simulink model "xmc_fir_import"  (R2023a)
settings: Solver=VariableStepAuto  StartTime=0.0  StopTime=inf  RelTol=1e-3
PostLoadFcn:
  | xmcHubUpdateInstalledDevice(gcs);
undefined symbols (not defined in the file): xc7vx485tffg1157
libraries: vmcUtilities x2, hlsBasic x2, dspsrcs4 x1, fir_c_import x1
settings Model: Creator=abehbood  LastModifiedBy=robg
settings SolverCC: AlgebraicLoopSolver=TrustRegion
settings DataIOCC: ReturnWorkspaceOutputs=off
settings OptimizationCC: LifeSpan=inf
settings DebuggingCC: UnconnectedInputMsg=warning  UnconnectedOutputMsg=warning  UnconnectedLineMsg=warning  ArithmeticOperatorsInVariantConditions=warning
settings ModelReferenceCC: EnableRefExpFcnMdlSchedulingChecks=on
settings SFSimCC: SimUseLocalCustomCode=off  CustomCodeUndefinedFunction=UseInterfaceOnly
settings RTWCC: RTWUseLocalCustomCode=off  DLArmComputeVersion=19.05
settings CodeAppCC: StateflowObjectComments=on

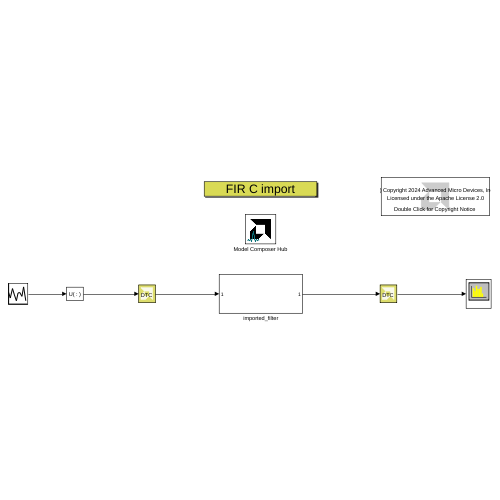
[thumbnail: Simulink's stored preview of the top-level diagram]
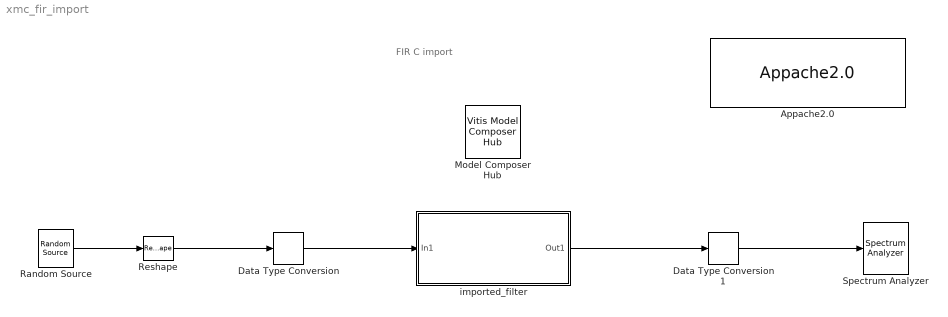
== system xmc_fir_import ==
  note: FIR C import
  Appache2.0 : vmcUtilities/Appache2.0
  Data Type Conversion : hlsBasic/Data Type Conversion  OutDataType=fixed  TypeExp=''  Signedness=Signed  WordLength=17  FractionalLength=14  RoundingMode=Truncation to minus infinity  OverflowMode=Wrap around
  Data Type Conversion1 : hlsBasic/Data Type Conversion  OutDataType=double  TypeExp=''  Signedness=Signed  WordLength=16  FractionalLength=0  RoundingMode=Truncation to minus infinity  OverflowMode=Wrap around
  Model Composer Hub : vmcUtilities/Vitis Model Composer Hub  Tag=genX  CodeGeneration=off  SubsystemName=imported_filter  StartColumn=1  NumberOfColumns=1  TargetDirectory=./code  exportDesign=off  analyzeDesign=off  validateDesignOnHw=off  ExportType=HLS C++ code  IpVendor=xilinx.com  IpLibrary=hls  IpVersion=1.0  IpHWLanguage=Verilog  AieCompilerOptions={}  AieSimulatorOptions={}  CreateTestbench=off  TestbenchStackSize=10  RunRtlSim=off  RunCSim=off  RunAieSim=off  AieSimTimeout=50000  RunAieSimProfiling=off  LaunchVitisAnalyzer=off  PlotOutput=off  RunX86Sim=on  X86SimTimeout=10  GenHwImage=off  GenLibadfXo=off  GenHwValidationCode=off  PlatformType=Not Specified  HwSystemType=Baremetal  HwValidationTarget=hw  ProjDevice=xc7vx485tffg1157-1  ProjDevicePart=xc7vx485tffg1157-1  SamplePeriod=-1  ClockFrequency=200  DataPathParallelism=1  xilinxfamily=Kintex7  part=xc7k325t  speed=-3  package=fbg676  directory=./netlist  testbench=off  incr_netlist=off  synthesis_tool=Vivado  clock_wrapper=Clock Enables  dbl_ovrd=According to Block Masks  dcm_input_clock_period=10  sysclk_period=10  simulink_period=1  eval_field=0  LogFileName=''  NThreads=4
  Random Source : dspsrcs4/Random Source  SrcType=Gaussian  NormMethod=Ziggurat  CltLength=12  MinVal=0  MaxVal=1  MeanVal=0  VarVal=1  RepMode=Not repeatable  rawSeed=1  IsInherit=off  SampMode=Discrete  SampTime=1  SampFrame=100  DataType=Double  OutComplex=Real  OutputFrames=off
  Reshape : Reshape
  Spectrum Analyzer : SpectrumAnalyzer  WindowPosition=[506 197 832 446]  Method=Welch  SampleRate=1  Span=1  StartFrequency=-0.5  StopFrequency=0.5  AveragingMethod=Exponential  YLimits=[-112.1969,21.3448]  ChannelNames="[\"\"]"  DefaultConfigurationName=spbscopes.SpectrumAnalyzerBlockCfg
  imported_filter : Subsystem
  wires:
  Data Type Conversion1/1 -> Spectrum Analyzer/1
  Random Source/1 -> Reshape/1
  Data Type Conversion/1 -> imported_filter/1(In1)
  imported_filter/1(Out1) -> Data Type Conversion1/1
  Reshape/1 -> Data Type Conversion/1

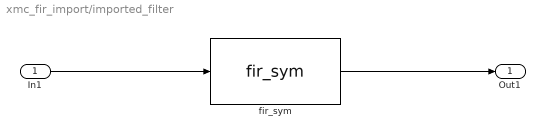
== system xmc_fir_import/imported_filter ==
  In1 : Inport
  fir_sym : fir_c_import/fir_sym  LibraryFunction=fir_sym  IncludeFiles={'fir_sym.h'}  SourceFiles={'fir.h', 'fir_sym.cpp', 'coef_halfof103.inc'}  IncludeDirectories={}  TemplateParams={' '}  FunctionParamTypes={xmcDataType('void'); xmcDataType('ap_fixed<17, 3, AP_TRN, AP_WRAP>'); xmcDataType('ap_fixed<17, 3, AP_TRN, AP_WRAP>')}  FunctionParamPassbys={0.000000000000000000e+00; 0.000000000000000000e+00; 0.000000000000000000e+00}  FunctionParamDimensions={'1'; '[100]'; '[100]'}  FunctionParamNames={'return'; 'din'; 'dout'}  FunctionParamDir={0.000000000000000000e+00; 1.000000000000000000e+00; 2.000000000000000000e+00}  FunctionParamSupportsStreaming={true; true; true}  BufferDepth={'0'}  FunctionParamValues={'0'; '0'; '0'}  ThroughputFactors={''}
  Out1 : Outport
  wires:
  In1/1 -> fir_sym/1
  fir_sym/1 -> Out1/1
